simulink model "PPU_NN"  (R2026a)
settings: Solver=FixedStepAuto  FixedStep=0.005  EnableMultiTasking=on
model workspace (MAT data in the model file):
  K_cte_forward_PPU = 1
  K_cte_reverse_PPU = 0.25
  L_AXLE_DIST_PPU = 3
  Lateral.xWheelbase.Value = 3
  Lateral.xWheelbase.Units = 'm'
  Lateral.xWheelbase.Comments = 'Wheelbase of the vehicle'
  Lateral.aMaxSteer.Value = 35
  Lateral.aMaxSteer.Units = 'deg'
  Lateral.aMaxSteer.Comments = ''
  Lateral.fSteerCutoff.Value = 314.159265
  Lateral.fSteerCutoff.Units = 'rad/s'
  Lateral.Stanley.NForward.Value = 1
  Lateral.Stanley.NReverse.Value = 0.25
  Lateral.Stanley.Units = ''
  Lateral.Stanley.Comments = ''
  Lateral.Pursuit.kLookahead.Value = 3
  Lateral.Pursuit.xLookaheadMin.Value = 0.5
  Lateral.Pursuit.xLookaheadMin.Units = 'm'
  Lateral.Pursuit.xLookaheadMax.Value = 20
  Lateral.Pursuit.xLookaheadMax.Units = 'm'
  Lateral.Pursuit.nWeightHeadingErr.Value = 0.5
  Lateral.Pursuit.Units = ''
  Lateral.Pursuit.Comments = ''
  Lateral.class.Value = 'Stanley'
  Lateral.class.Units = ''
  Lateral.class.Comments = ''
  MAX_STEERING_ANGLE_DEG_PPU = 35
libraries: dspstat3 x5, procinterlib x2, deeplib x1
settings Model: Creator=lnicolet  LastModifiedBy=chmurski
settings SolverCC: PositivePriorityOrder=on
settings OptimizationCC: StrengthReduction=on  EfficientMapNaN2IntZero=off  MaxStackSize=2048
settings HardwareCC: ProdLargestAtomicInteger=Long  ProdHWDeviceType=Infineon->PPU  TargetLargestAtomicInteger=Long  TargetLargestAtomicFloat=Float  TargetLongLongMode=on  TargetIntDivRoundTo=Zero  TargetEndianess=LittleEndian  TargetHWDeviceType=Infineon->PPU  HardwareBoardFeatureSet=SoCBlockset
settings ModelReferenceCC: ModelReferenceNumInstancesAllowed=Single
settings RTWCC: SystemTargetFile=ert.tlc  HardwareBoard=Infineon AURIX TC4x  TLCOptions=-aInlineSetEventsForThisBaseRateFcn=TLC_FALSE -aSuppressMultiTaskScheduler=TLC_FALSE -aRateBasedStepFcn=1  RetainRTWFile=on  Toolchain=Synopsys(R) MetaWare for Infineon AURIX TC4x  BuildConfiguration=Specify  Description=Embedded Coder
settings CodeAppCC: MaxIdLength=256.0
settings ERTTargetCC: ExtModeTransport=3.0  ERTFilePackagingFormat=Compact  DynamicArrayContainerType=coder::array  CodeReplacementLibrary=MetaWare TC4x PPU DSPLib,MetaWare TC4x PPU Veclib  SuppressErrorStatus=on

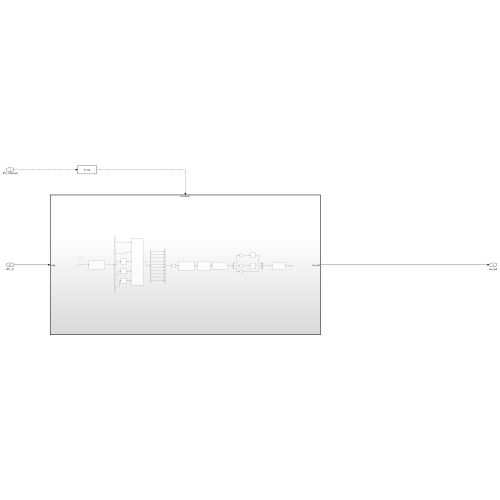
[thumbnail: Simulink's stored preview of the top-level diagram]
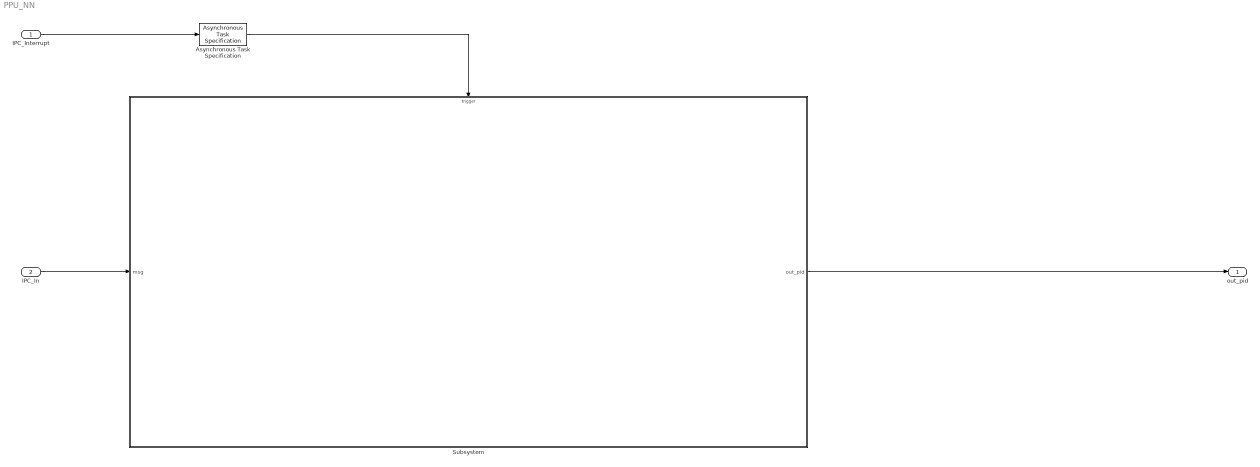
== system PPU_NN ==
  IPC_Interrupt : Inport  OutputFunctionCall=on
  IPC_In : Inport  Port=2
  Asynchronous Task Specification : AsynchronousTaskSpecification  TaskPriority=50
  Subsystem : Subsystem  TreatAsAtomicUnit=on
  out_pid : Outport
  wires:
  Subsystem/1(out_pid) -> out_pid/1
  IPC_In/1 -> Subsystem/1(msg)
  Asynchronous Task Specification/1 -> Subsystem/Trigger
  IPC_Interrupt/1 -> Asynchronous Task Specification/1

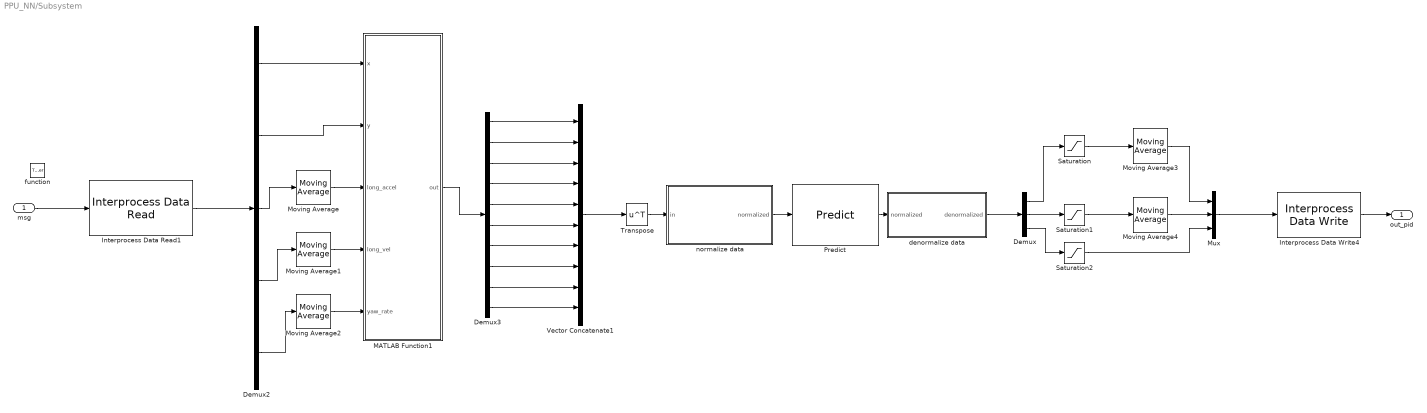
== system PPU_NN/Subsystem ==
  msg : Inport
  function : TriggerPort  TriggerType=function-call  VariantControl=(inherit)
  Demux : Demux  Outputs=3
  Demux2 : Demux  Outputs=[5,5,1,1,1]
  Demux3 : Demux  Outputs=10
  Interprocess Data Read1 : procinterlib/Interprocess Data Read  showPort=on  DataType=single  NumBuffers=1  DataLength=13  ChannelNum=0  IsIntEnabled=1  EnInterrupt=off  StructForBus=struct( 'signal1', uint16( 0 ), 'signal2', uint16( 0 ) )  IPCBetween=5  CurrentPU=6  PartCores=TriCore0<->PPU  SampleTime=-1  TargetType=1  ClientPU=TriCore0  ClientIntPrio=50  CurrentPUPriority=1
  Interprocess Data Write4 : procinterlib/Interprocess Data Write  showPort=on  ChannelNum=1  NumBuff=1  IsIntEnabled=0  EnInterrupt=off  IPCBetween=5  CurrentPU=6  DataType=single  PartCores=TriCore0<->PPU  TargetType=1  ClientPU=TriCore0  ClientIntPrio=45  CurrentPUPriority=1
      settings: LibrarySourceBlock=c2000lib/Target Communication/Interprocess Data Write
  MATLAB Function1 : MATLAB Function  TreatAsAtomicUnit=on
  Moving Average{,1..4} (5 alike) : dspstat3/Moving Average  Method=Sliding window  ForgettingFactorPort=off  SpecifyWindowLength=on  WindowLengthSource=Property  MaxWindowLength=20  WindowLength=50  OverlapLength=49  AllowArbitraryInputLength=off  ForgettingFactor=0.9  SimulateUsing=Interpreted execution
  Mux : Mux  Inputs=3
  Predict : deeplib/Predict  Network=Network from MAT-file  NetworkFunction=squeezenet  NetworkFilePath=.\trained_pid_network.mat  MiniBatchSize=1  SimulateUsing=Auto mode  InputDataFormats={'',''}  Predictions=on  Activations={}  ForceInterpretedSim=off  EnableDLNetwork=on  LastKnownNetworkFilePath=''  LastKnownNetworkTimeStamp=''
      link override "MLFB/ Demux ": Outputs=1
      link override "MLFB/ SFunction ": FunctionName=sf_sfun
      link override MLFB/in_1: Port=1
      link override MLFB/out_1_predict: Port=1
  Saturation : Saturate  UpperLimit=25  LowerLimit=12
  Saturation1 : Saturate  UpperLimit=0.05  LowerLimit=0
  Saturation2 : Saturate  UpperLimit=2  LowerLimit=1.99
  Transpose : Math  Operator=transpose
  Vector Concatenate1 : Concatenate  NumInputs=10
  denormalize data : MATLAB Function  TreatAsAtomicUnit=on
  normalize data : MATLAB Function  TreatAsAtomicUnit=on
  out_pid : Outport
  wires:
  msg/1 -> Interprocess Data Read1/1
  Interprocess Data Write4/1 -> out_pid/1
  Predict/1 -> denormalize data/1(normalized)
  Transpose/1 -> normalize data/1(in)
  Demux3/7 -> Vector Concatenate1/7
  Demux3/10 -> Vector Concatenate1/10
  Demux3/3 -> Vector Concatenate1/3
  Demux3/9 -> Vector Concatenate1/9
  Demux3/4 -> Vector Concatenate1/4
  Moving Average1/1 -> MATLAB Function1/4(long_vel)
  MATLAB Function1/1(out) -> Demux3/1
  Moving Average2/1 -> MATLAB Function1/5(yaw_rate)
  Demux3/1 -> Vector Concatenate1/1
  Demux3/5 -> Vector Concatenate1/5
  Demux3/6 -> Vector Concatenate1/6
  Demux3/2 -> Vector Concatenate1/2
  Moving Average/1 -> MATLAB Function1/3(long_accel)
  Demux3/8 -> Vector Concatenate1/8
  Vector Concatenate1/1 -> Transpose/1
  Interprocess Data Read1/1 -> Demux2/1
  normalize data/1(normalized) -> Predict/1
  denormalize data/1(denormalized) -> Demux/1
  Mux/1 -> Interprocess Data Write4/1
  Demux/1 -> Saturation/1
  Demux/2 -> Saturation1/1
  Demux/3 -> Saturation2/1
  Saturation/1 -> Moving Average3/1
  Saturation1/1 -> Moving Average4/1
  Saturation2/1 -> Mux/3
  Moving Average3/1 -> Mux/1
  Moving Average4/1 -> Mux/2
  Demux2/1 -> MATLAB Function1/1(x)
  Demux2/2 -> MATLAB Function1/2(y)
  Demux2/3 -> Moving Average/1
  Demux2/4 -> Moving Average1/1
  Demux2/5 -> Moving Average2/1

== matlab function PPU_NN/Subsystem/MATLAB Function1 ==
  data: x input; y input; long_accel input; long_vel input; yaw_rate input; out output size=[1,10]
function out = fcn(x, y, long_accel, long_vel, yaw_rate)
% x, y       - buffered last 50 coordinates
% long_accel - mean value over last 50 samples
% long_vel   - mean value over last 50 samples
% yaw_rate   - mean value over last 50 samples

    % calculate the coefficients
    % coeffs = [0,0,0,0,0,0,0];
    coeffs = polyfit(x, y, 6);


    %out = [coeffs, 0,0,0, long_accel, long_vel, yaw_rate];
    out = [coeffs, long_accel, long_vel, yaw_rate];
end

== matlab function PPU_NN/Subsystem/denormalize data ==
  data: normalized input; denormalized output
function denormalized = denormalize_data(normalized)
means = [16.877973565397809,0.180179969890152,2];
stds = [3.766904692168230,0.227742668578153,1];

denormalized = normalized .* stds + means;
%denormalized = denormalized';

== matlab function PPU_NN/Subsystem/normalize data ==
  data: in input; normalized output
function normalized = normalize_data(in)

means = [-4.637948169071871e-06,-0.001860122528536,-1.253301709668094,-2.670191808853602e+02,-3.691746945912067e+04,-2.604027473248851e+06,-7.753576608458824e+07,-0.026465574971934,12.001809631893268,0.543761765148791];
% overriding zero standard deviation of the first feature to prevent zero division
%stds = 1.0e+03 * [0.0243, 1.2462, 30.5869, 344.1872, 1.4759e+03, 1, 4.9778, 2.2616, 0.7889, 1.0174];
stds = [0.003207066660745,1.120617980438591,2.898147742492388e+02,6.305005554713097e+04,8.330388422937828e+06,5.909552153813827e+08,1.747622542352282e+10,0.205339470500643,0.883106632297858,1.828250162966217];

normalized = (in - means) ./ stds;
